simulink model "recursive_gru_update"  (R2020a)
settings: Solver=FixedStepAuto  StartTime=449  StopTime=497  FixedStep=1  RelTol=1e-3
undefined symbols (not defined in the file or in its folder): mu, sigma
settings Model: Creator=tyoshida  LastModifiedBy=tyoshida
settings DataIOCC: ExternalInput=[TimeData, SimInVariables]  LoadExternalInput=on

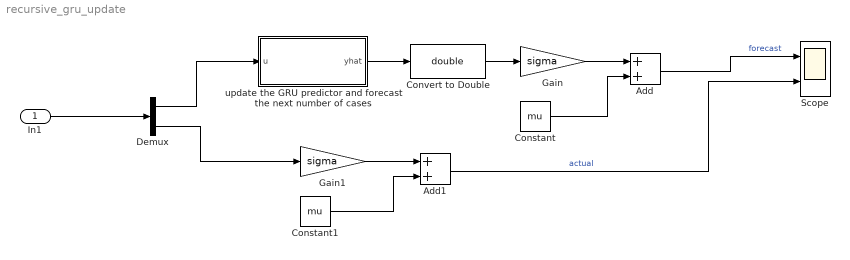
== system recursive_gru_update ==
  In1 : Inport  PortDimensions=2
  Add : Sum
  Add1 : Sum
  Constant : Constant  Value=mu
  Constant1 : Constant  Value=mu
  Convert to Double : DataTypeConversion  OutDataTypeStr=double
  Demux : Demux  Outputs=2
  Gain : Gain  Gain=sigma
  Gain1 : Gain  Gain=sigma
  Scope : Scope  NumInputPorts=2
  "update the GRU predictor and forecast the next number of cases  " : MATLAB Function  TreatAsAtomicUnit=on
  wires:
  Gain/1 -> Add/1
  Constant/1 -> Add/2
  Add/1 -> Scope/1  "forecast"
  In1/1 -> Demux/1
  Demux/1 -> "update the GRU predictor and forecast the next number of cases  "/1(u)
  Constant1/1 -> Add1/2
  Add1/1 -> Scope/2  "actual"
  Gain1/1 -> Add1/1
  Demux/2 -> Gain1/1
  "update the GRU predictor and forecast the next number of cases  "/1(yhat) -> Convert to Double/1
  Convert to Double/1 -> Gain/1

== matlab function recursive_gru_update/update the GRU predictor and forecast the next number of cases   ==
  data: u input; yhat output
function yhat = GRU_Predicotr(u)

yhat = single(0); % WA because the analyzer cannot identify this data type for code generation

coder.extrinsic('my_update_predict_fcn'); % declare extrinsic functions for code generation

yhat = my_update_predict_fcn(u);
